simulink model "per_ut"  (Simulink 8.1)
settings: Solver=FixedStepDiscrete  StartTime=0.0  StopTime=10.0  FixedStep=0.005  RelTol=1e-3
PostLoadFcn:
  | , if any(exist('dsrtsu_mdlpostloadfcn', 'file') == [2, 3, 6]), try dsrtsu_mdlpostloadfcn('Execute', bdroot); catch fprintf('Error in PostLoadFcn (dsrtsu_mdlpostloadfcn) for model "%s":\n %s\n', bdroot, lasterr); end, end,
undefined symbols (not defined in the file or in its folder): VDINR_CamFailsafeMode_flg, VDINR_CamImageStatus_enum, VDINR_CamInternalError_flg, VDINR_RadCurrentPower_enum, VDINR_RadRxInvalid_enum, VDINR_RadSensorBlockage_flg, VDINR_RadSensorDefective_flg, VDINR_RadSensTempErr_flg, VDINR_RadSupplyVoltLow_flg, VMOT_NOFTRACKS_num, VMOT_TRACKSOBST_enum, VMOT_TRACKSVEL_mps, VMOT_TRACKSWIDTH_m, VMOT_TRACKSX_m, VMOT_TRACKSY_m
libraries: siltestlib x24, simulink x1, per x1
settings Model: DSRTSU_INTERNAL_RTI_VER=450  DSRTSU_INTERNAL_RTI_TYPE=rti1401  RTICANMMDATA=struct('GeneralSetupData',struct('modelroot','D:\Soichi\SVNDATA\haitec_adas\Phase2\trunk\Application\AdasDragon\software\sw_development\arch\app\per','generalsettings',struct('filesettings',struct('destfolder',struct('Name','RTICANMM_FILES','Check',1),'buildfolder',struct('Name','.','Check',1),'AbsDestfolder',struct('Name','D:\Soichi\SVNDATA\haitec_adas\Phase2\trunk\Application\AdasDragon\software\sw_development\arch\app\per\RTICANMM_FILES'),'AbsBuildfolder',struct('Name','D:\Soichi\SVNDATA\haitec_adas\Phase2\trunk\Application\AdasDragon\software\sw_development\arch\app\per'))),'options',struct('addpaths',1,'rmpaths',1,'addtrcexclusion',logical(1),'cannavigator',struct('checkmonitoring',0),'show_usrtrc',0,'use_usrtrc',0),'advanced',struct('options',[1 1 1 1 1 1 1 1 1 1 1 1 1 1 1 1 1 1 1 1 1 1 1 1 1 1 1 1 1 1 1 1 1 1 1 1 1 1 1 1 1 1 1 1 1 1 1 1 1 1 1 1 1 1 1 1 1 1 1 1 1 1 1 1 1 1 1 1 1 1 1 1 1 1 1 1 1 1 1 1 1 1 1 1 1 1 1 1 1 1 1 1 1 1 1 1 1 1 1 1]),'MPSetup',{{}},'modelname','per_ut','block','per_ut'))  DSRTSU_INTERNAL_RTIFPGA=40  Creator=xsellart  LastModifiedBy=AT015411
settings DataIOCC: SignalLoggingSaveFormat=Dataset
settings OptimizationCC: ExpressionDepthLimit=128
settings DebuggingCC: FcnCallInpInsideContextMsg=EnableAllAsError
settings HardwareCC: ProdIntDivRoundTo=Zero  ProdEndianess=BigEndian  ProdHWDeviceType=Generic->Custom  TargetIntDivRoundTo=Zero  TargetEndianess=BigEndian  TargetHWDeviceType=Generic->Custom
settings RTWCC: SystemTargetFile=rti1401.tlc  MakeCommand=make_rti  TemplateMakefile=rti1401.tmf  Description=dSPACE DS1401 Hardware Platform  ProcessScript=rti1401_make_rtw_hook
settings STFCustomTargetCC: CodeReplacementLibrary=ANSI_C  ParMdlRefBuildCompliant=on  GeneratePreprocessorConditionals=Disable all  SystemTargetFile=rti1401.tlc
settings GRTTargetCC: CompOptLevelCompliant=off  ConcurrentExecutionCompliant=off  MatFileLogging=off  ExtModeMexFile=noextcomm
settings CustomProperty: DataType=RTWOptions_EnumType_D__Program Files_dSPACE RCPHIL 2014-B_MATLAB_RTI_RTI1401_TLC_rti1401_1InitialSimState  Value=RUN
settings EnumStrPairs: String=RUN

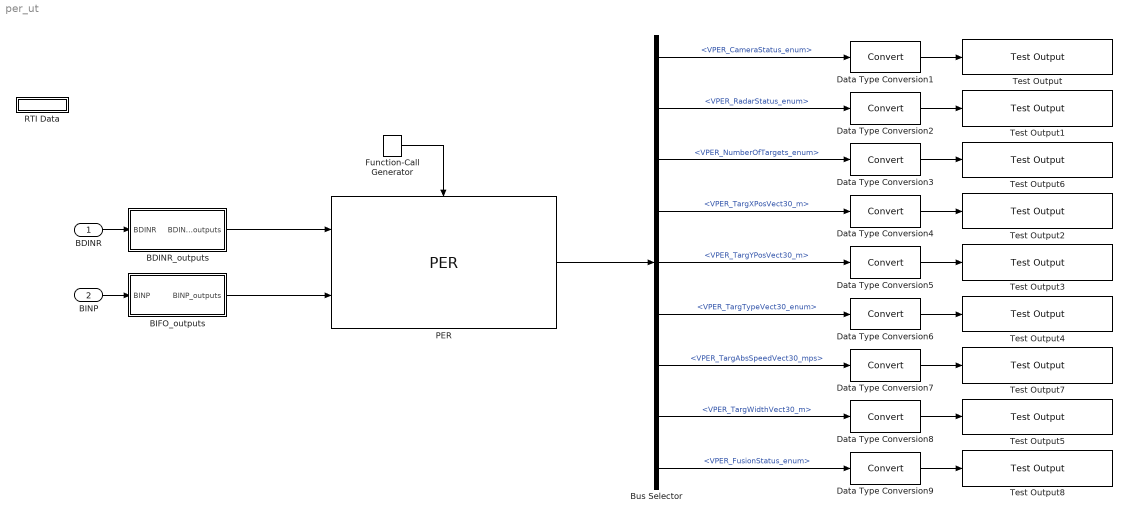
== system per_ut ==
  BDINR : Inport  OutDataTypeStr=Bus: BDINR_outputs
  BINP : Inport  Port=2  OutDataTypeStr=Bus: BINP_outputs
  BDINR_outputs : Subsystem
  BIFO_outputs : Subsystem
  Bus Selector : BusSelector  OutputSignals=VPER_CameraStatus_enum,VPER_RadarStatus_enum,VPER_NumberOfTargets_enum,VPER_TargXPosVect30_m,VPER_TargYPosVect30_m,VPER_TargTypeVect30_enum,VPER_TargAbsSpeedVect30_mps,VPER_TargWidthVect30_m,VPER_FusionStatus_enum
  Data Type Conversion{1..9} (9 alike) : DataTypeConversion
  Function-Call Generator : simulink/Ports & Subsystems/Function-Call Generator  sample_time=1  numberOfIterations=1
  PER : per/PER
  RTI Data : Subsystem  Tag=struct('RTIDataServer',struct('RTIDataServerVs','2','RTIModelDescription','struct(''main'',''per_ut'',''sub'','''',''isMp'',0)'))  LoadFcn="if exist('rtidc'), try,  rtidc('DataHostBlockClbLoad', gcbh); catch, disp(['Warning: ''LoadFcn'' for RTI Data block failed: ' lasterr]); end, end,"  mask(RTI_DATA_HOST){}
      mask help:
      | RTI Data Block.
      | This block is used by RTI to store internal model-dependent data.
      | Please keep this block on the root level of the model. Deleting this block will result in data loss.
      |
      | NEVER DELETE OR COPY THIS BLOCK!
      settings: CopyFcn="if exist('rtidc'), try,  rtidc('DataHostBlockClbCopy', gcbh); catch, disp(['Warning: ''CopyFcn'' for RTI Data block failed: ' lasterr]); end, end,"  DeleteFcn="if exist('rtidc'), try,  rtidc('DataHostBlockClbDelete', gcbh); catch, disp(['Warning: ''DeleteFcn'' for RTI Data block failed: ' lasterr]); end, end,"  ModelCloseFcn="if exist('rtidc'), try,  rtidc('DataHostBlockClbModelClose', gcbh); catch, disp(['Warning: ''ModelCloseFcn'' for RTI Data block failed: ' lasterr]); end, end,"  PreSaveFcn="if exist('rtidc'), try,  rtidc('DataHostBlockClbPreSave', gcbh); catch, disp(['Warning: ''PreSaveFcn'' for RTI Data block failed: ' lasterr]); end, end,"  PostSaveFcn="if exist('rtidc'), try,  rtidc('DataHostBlockClbPostSave', gcbh); catch, disp(['Warning: ''PostSaveFcn'' for RTI Data block failed: ' lasterr]); end, end,"  NameChangeFcn="if exist('rtidc'), try,  rtidc('DataHostBlockClbNameChange', gcbh); catch, disp(['Warning: ''NameChangeFcn'' for RTI Data block failed: ' lasterr]); end, end,"
      mask Help:
      | RTI Data Block.
      | This block is used by RTI to store internal model-dependent data.
      | Please keep this block on the root level of the model. Deleting this block will result in data loss.
      | 
      | NEVER DELETE OR COPY THIS BLOCK!
      mask Display:
      | text(0.5, 0.5, 'RTI Data', 'HorizontalAlignment', 'center');
      | plot([1 0]);
  Test Output : siltestlib/Test Output  varname=VPER_CameraStatus_enum  sampletime=-1
  Test Output1 : siltestlib/Test Output  varname=VPER_RadarStatus_enum  sampletime=-1
  Test Output2 : siltestlib/Test Output  varname=VPER_TargXPosVect30_m  sampletime=-1
  Test Output3 : siltestlib/Test Output  varname=VPER_TargYPosVect30_m  sampletime=-1
  Test Output4 : siltestlib/Test Output  varname=VPER_TargTypeVect30_enum  sampletime=-1
  Test Output5 : siltestlib/Test Output  varname=VPER_TargWidthVect30_m  sampletime=-1
  Test Output6 : siltestlib/Test Output  varname=VPER_NumberOfTargets_enum  sampletime=-1
  Test Output7 : siltestlib/Test Output  varname=VPER_TargAbsSpeedVect30_mps  sampletime=-1
  Test Output8 : siltestlib/Test Output  varname=VPER_FusionStatus_enum  sampletime=-1
  wires:
  BDINR_outputs/1(BDINR_outputs) -> PER/1
  BIFO_outputs/1(BINP_outputs) -> PER/2
  BDINR/1 -> BDINR_outputs/1(BDINR)
  BINP/1 -> BIFO_outputs/1(BINP)
  Function-Call Generator/1 -> PER/Trigger
  Bus Selector/1 -> Data Type Conversion1/1  "<VPER_CameraStatus_enum>"
  Data Type Conversion1/1 -> Test Output/1
  Bus Selector/2 -> Data Type Conversion2/1  "<VPER_RadarStatus_enum>"
  Data Type Conversion2/1 -> Test Output1/1
  Bus Selector/3 -> Data Type Conversion3/1  "<VPER_NumberOfTargets_enum>"
  Data Type Conversion4/1 -> Test Output2/1
  Bus Selector/4 -> Data Type Conversion4/1  "<VPER_TargXPosVect30_m>"
  Data Type Conversion5/1 -> Test Output3/1
  Bus Selector/5 -> Data Type Conversion5/1  "<VPER_TargYPosVect30_m>"
  Data Type Conversion6/1 -> Test Output4/1
  Bus Selector/6 -> Data Type Conversion6/1  "<VPER_TargTypeVect30_enum>"
  Data Type Conversion8/1 -> Test Output5/1
  PER/1 -> Bus Selector/1
  Bus Selector/7 -> Data Type Conversion7/1  "<VPER_TargAbsSpeedVect30_mps>"
  Data Type Conversion3/1 -> Test Output6/1
  Bus Selector/8 -> Data Type Conversion8/1  "<VPER_TargWidthVect30_m>"
  Data Type Conversion7/1 -> Test Output7/1
  Data Type Conversion9/1 -> Test Output8/1
  Bus Selector/9 -> Data Type Conversion9/1  "<VPER_FusionStatus_enum>"

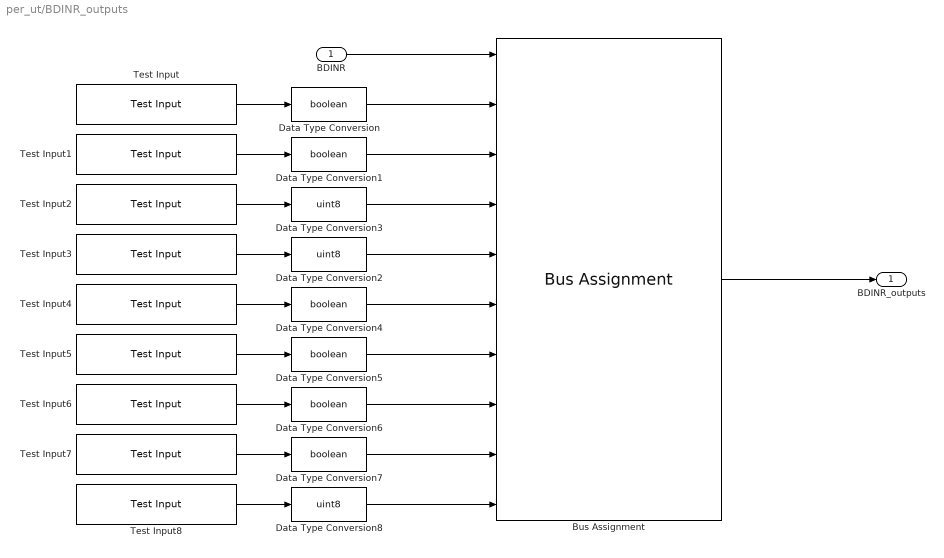
== system per_ut/BDINR_outputs ==
  BDINR : Inport  OutDataTypeStr=Bus: BDINR_outputs
  Bus Assignment : BusAssignment  AssignedSignals=VDINR_CamInternalError_flg,VDINR_CamFailsafeMode_flg,VDINR_CamImageStatus_enum,VDINR_RadRxInvalid_enum,VDINR_RadSupplyVoltLow_flg,VDINR_RadSensorDefective_flg,VDINR_RadSensorBlockage_flg,VDINR_RadSensTempErr_flg,VDINR_RadCurrentPower_enum
  Data Type Conversion{,1,4..7} (6 alike) : DataTypeConversion  OutDataTypeStr=boolean
  Data Type Conversion2 : DataTypeConversion  OutDataTypeStr=uint8
  Data Type Conversion3 : DataTypeConversion  OutDataTypeStr=uint8
  Data Type Conversion8 : DataTypeConversion  OutDataTypeStr=uint8
  Test Input : siltestlib/Test Input  varname=VDINR_CamInternalError_flg  sampletime=-1
  Test Input1 : siltestlib/Test Input  varname=VDINR_CamFailSafeMode_flg  sampletime=-1
  Test Input2 : siltestlib/Test Input  varname=VDINR_CamImageStatus_enum  sampletime=-1
  Test Input3 : siltestlib/Test Input  varname=VDINR_RadRxInvalid_enum  sampletime=-1
  Test Input4 : siltestlib/Test Input  varname=VDINR_RadSupplyVoltLow_flg  sampletime=-1
  Test Input5 : siltestlib/Test Input  varname=VDINR_RadSensorDefective_flg  sampletime=-1
  Test Input6 : siltestlib/Test Input  varname=VDINR_RadSensorBlockage_flg  sampletime=-1
  Test Input7 : siltestlib/Test Input  varname=VDINR_RadSensTempErr_flg  sampletime=-1
  Test Input8 : siltestlib/Test Input  varname=VDINR_RadCurrentPower_enum  sampletime=-1
  BDINR_outputs : Outport  OutDataTypeStr=Bus: BDINR_outputs
  wires:
  Bus Assignment/1 -> BDINR_outputs/1
  BDINR/1 -> Bus Assignment/1
  Test Input/1 -> Data Type Conversion/1
  Data Type Conversion/1 -> Bus Assignment/2
  Test Input1/1 -> Data Type Conversion1/1
  Data Type Conversion1/1 -> Bus Assignment/3
  Test Input2/1 -> Data Type Conversion3/1
  Data Type Conversion3/1 -> Bus Assignment/4
  Test Input3/1 -> Data Type Conversion2/1
  Data Type Conversion2/1 -> Bus Assignment/5
  Test Input4/1 -> Data Type Conversion4/1
  Data Type Conversion4/1 -> Bus Assignment/6
  Test Input5/1 -> Data Type Conversion5/1
  Data Type Conversion5/1 -> Bus Assignment/7
  Test Input6/1 -> Data Type Conversion6/1
  Data Type Conversion6/1 -> Bus Assignment/8
  Test Input7/1 -> Data Type Conversion7/1
  Data Type Conversion7/1 -> Bus Assignment/9
  Test Input8/1 -> Data Type Conversion8/1
  Data Type Conversion8/1 -> Bus Assignment/10

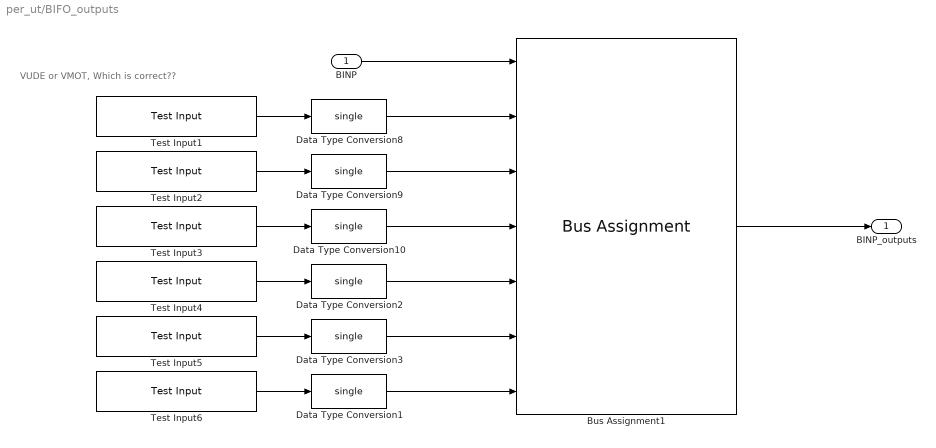
== system per_ut/BIFO_outputs ==
  note: VUDE or VMOT, Which is correct??
  BINP : Inport  OutDataTypeStr=Bus: BINP_outputs
  Bus Assignment1 : BusAssignment  AssignedSignals=VMOT_NOFTRACKS_num,VMOT_TRACKSX_m,VMOT_TRACKSY_m,VMOT_TRACKSOBST_enum,VMOT_TRACKSVEL_mps,VMOT_TRACKSWIDTH_m
  Data Type Conversion{1..3,8..10} (6 alike) : DataTypeConversion  OutDataTypeStr=single
  Test Input1 : siltestlib/Test Input  varname=VUDE_NOfTracks_num  sampletime=-1
  Test Input2 : siltestlib/Test Input  varname=VUDE_TracksX_num  sampletime=-1
  Test Input3 : siltestlib/Test Input  varname=VUDE_TracksY_num  sampletime=-1
  Test Input4 : siltestlib/Test Input  varname=VUDE_TracksObsType_num  sampletime=-1
  Test Input5 : siltestlib/Test Input  varname=VUDE_TracksVel_mps  sampletime=-1
  Test Input6 : siltestlib/Test Input  varname=VUDE_TracksWidth_enum  sampletime=-1
  BINP_outputs : Outport  OutDataTypeStr=Bus: BINP_outputs
  wires:
  BINP/1 -> Bus Assignment1/1
  Bus Assignment1/1 -> BINP_outputs/1
  Test Input1/1 -> Data Type Conversion8/1
  Data Type Conversion8/1 -> Bus Assignment1/2
  Test Input2/1 -> Data Type Conversion9/1
  Data Type Conversion9/1 -> Bus Assignment1/3
  Test Input3/1 -> Data Type Conversion10/1
  Data Type Conversion10/1 -> Bus Assignment1/4
  Test Input4/1 -> Data Type Conversion2/1
  Data Type Conversion2/1 -> Bus Assignment1/5
  Test Input5/1 -> Data Type Conversion3/1
  Data Type Conversion3/1 -> Bus Assignment1/6
  Test Input6/1 -> Data Type Conversion1/1
  Data Type Conversion1/1 -> Bus Assignment1/7

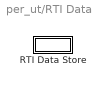
== system per_ut/RTI Data ==
  RTI Data Store : Subsystem  Tag=struct('private',struct('version',struct('dsVer',uint32(2),'dsVerCreation',uint32(2),'RTI',struct('ver','7.3','type','RTI1401')),'access',struct('type','Model','isPerm',1,'created',['28-Oct-2015 16:09:34'],'modified',['26-Nov-2015 15:58:00'],'location','')),'public',struct('main',struct('data',[]),'sub',struct('name','','data',[])))  mask(RTI_DATA_STORE){}
      mask help:
      | RTI Data Store Block. This block is used by RTI to store internal model dependent data. Deleting this block will result in data loss.
      |
      | NEVER DELETE, COPY, OR MODIFY THIS BLOCK!
      mask Help:
      | RTI Data Store Block. This block is used by RTI to store internal model dependent data. Deleting this block will result in data loss.
      | 
      | NEVER DELETE, COPY, OR MODIFY THIS BLOCK!
      mask Display: text(0.5, 0.5, ' ', 'HorizontalAlignment', 'center');

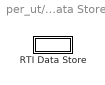
== system per_ut/RTI Data/RTI Data Store ==
  RTI Data Store : Subsystem  mask(RTI_DATA_STORE){}
      mask help:
      | RTI Data Store Block. This block is used by RTI to store internal model dependent data. Deleting this block will result in data loss.
      |
      | NEVER DELETE, COPY, OR MODIFY THIS BLOCK!
      mask Help:
      | RTI Data Store Block. This block is used by RTI to store internal model dependent data. Deleting this block will result in data loss.
      | 
      | NEVER DELETE, COPY, OR MODIFY THIS BLOCK!
      mask Display: text(0.5, 0.5, ' ', 'HorizontalAlignment', 'center');

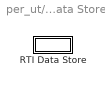
== system per_ut/RTI Data/RTI Data Store/RTI Data Store ==
  RTI Data Store : Subsystem  mask(RTI_DATA_STORE){}
      mask help:
      | RTI Data Store Block. This block is used by RTI to store internal model dependent data. Deleting this block will result in data loss.
      |
      | NEVER DELETE, COPY, OR MODIFY THIS BLOCK!
      mask Help:
      | RTI Data Store Block. This block is used by RTI to store internal model dependent data. Deleting this block will result in data loss.
      | 
      | NEVER DELETE, COPY, OR MODIFY THIS BLOCK!
      mask Display: text(0.5, 0.5, ' ', 'HorizontalAlignment', 'center');

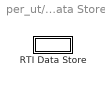
== system per_ut/RTI Data/RTI Data Store/RTI Data Store/RTI Data Store ==
  RTI Data Store : Subsystem  mask(RTI_DATA_STORE){}
      mask help:
      | RTI Data Store Block. This block is used by RTI to store internal model dependent data. Deleting this block will result in data loss.
      |
      | NEVER DELETE, COPY, OR MODIFY THIS BLOCK!
      mask Help:
      | RTI Data Store Block. This block is used by RTI to store internal model dependent data. Deleting this block will result in data loss.
      | 
      | NEVER DELETE, COPY, OR MODIFY THIS BLOCK!
      mask Display: text(0.5, 0.5, ' ', 'HorizontalAlignment', 'center');

== system per_ut/RTI Data/RTI Data Store/RTI Data Store/RTI Data Store/RTI Data Store ==
